simulink model "debugGyros"  (Simulink 9.0)
settings: Solver=FixedStepDiscrete  StartTime=0.0  StopTime=inf  FixedStep=0.01  RelTol=1e-3  EnableMultiTasking=on
InitFcn:
  | ROBOT_DOF=23;
libraries: WBToolboxLibrary x9
settings Model: SuppressorTable=22 serialization::archive 11 0 6 0 0 0 11 0  Creator=DanielePucci  LastModifiedBy=icub
settings DataIOCC: LimitDataPoints=on  SaveFormat=StructureWithTime
settings DebuggingCC: UnderspecifiedInitializationDetection=Simplified  MergeDetectMultiDrivingBlocksExec=error
settings HardwareCC: ProdBitPerPointer=64  ProdLargestAtomicFloat=Float  ProdIntDivRoundTo=Zero  ProdEndianess=LittleEndian  ProdHWDeviceType=Specified

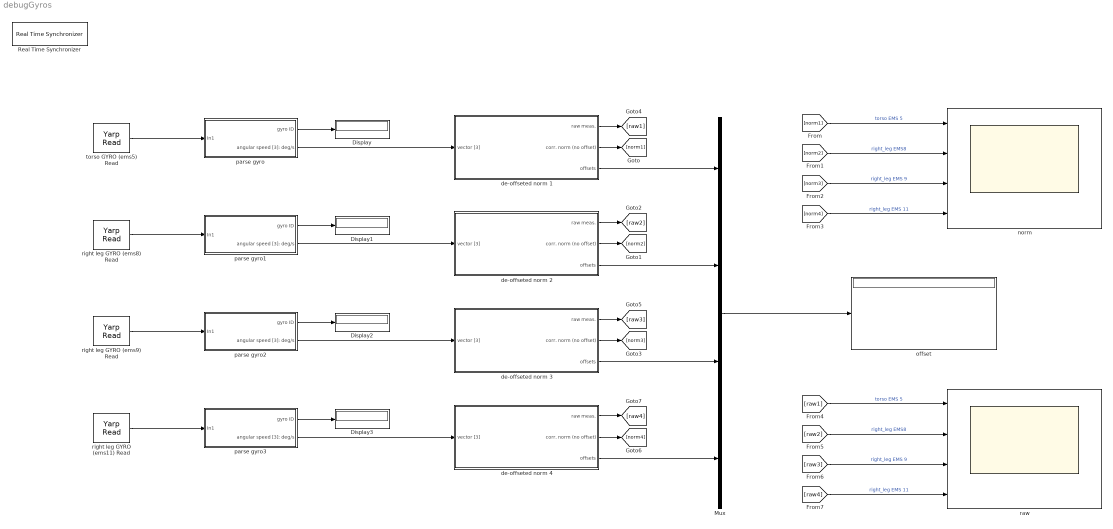
== system debugGyros ==
  Display{,1..3} (4 alike) : Display
  Mux : Mux
  Real Time Synchronizer : WBToolboxLibrary/Utilities/Real Time Synchronizer  period=0.01
      settings: SourceProductName=Whole Body Toolbox
  de-offseted norm 1 : Subsystem
  de-offseted norm 2 : Subsystem
  de-offseted norm 3 : Subsystem
  de-offseted norm 4 : Subsystem
  "norm " : Scope  NumInputPorts=4
  offset : Display
  parse gyro : Subsystem
  parse gyro1 : Subsystem
  parse gyro2 : Subsystem
  parse gyro3 : Subsystem
  raw : Scope  NumInputPorts=4
  right leg GYRO (ems11) Read : WBToolboxLibrary/Utilities/Yarp Read  portName='/icub/right_leg/inertialMTB'  signalSize=86  blocking=off  timestamp=off  autoconnect=on  errorOnConnection=off
      settings: SourceProductName=Whole Body Toolbox
  right leg GYRO (ems8) Read : WBToolboxLibrary/Utilities/Yarp Read  portName='/icub/right_leg/inertialEMS8'  signalSize=8  blocking=off  timestamp=off  autoconnect=on  errorOnConnection=off
      settings: SourceProductName=Whole Body Toolbox
  right leg GYRO (ems9) Read : WBToolboxLibrary/Utilities/Yarp Read  portName='/icub/right_leg/inertialEMS9'  signalSize=8  blocking=off  timestamp=off  autoconnect=on  errorOnConnection=off
      settings: SourceProductName=Whole Body Toolbox
  torso GYRO (ems5) Read : WBToolboxLibrary/Utilities/Yarp Read  portName='/icub/torso/inertialEMS5'  signalSize=8  blocking=off  timestamp=off  autoconnect=on  errorOnConnection=off
      settings: SourceProductName=Whole Body Toolbox
  wires:
  torso GYRO (ems5) Read/1 -> parse gyro/1(In1)
  parse gyro/2(angular speed [3]: deg/s) -> de-offseted norm 1/1(vector [3])
  parse gyro1/2(angular speed [3]: deg/s) -> de-offseted norm 2/1(vector [3])
  right leg GYRO (ems8) Read/1 -> parse gyro1/1(In1)
  parse gyro2/2(angular speed [3]: deg/s) -> de-offseted norm 3/1(vector [3])
  right leg GYRO (ems9) Read/1 -> parse gyro2/1(In1)
  parse gyro3/2(angular speed [3]: deg/s) -> de-offseted norm 4/1(vector [3])
  right leg GYRO (ems11) Read/1 -> parse gyro3/1(In1)
  parse gyro/1(gyro ID) -> Display/1
  parse gyro1/1(gyro ID) -> Display1/1
  parse gyro2/1(gyro ID) -> Display2/1
  parse gyro3/1(gyro ID) -> Display3/1
  de-offseted norm 1/3(offsets) -> Mux/1
  de-offseted norm 2/3(offsets) -> Mux/2
  de-offseted norm 3/3(offsets) -> Mux/3
  de-offseted norm 4/3(offsets) -> Mux/4
  Mux/1 -> offset/1
  de-offseted norm 1/2(corr. norm (no offset)) -> [norm1]
  [norm1] -> "norm "/1  "torso EMS 5"
  [norm2] -> "norm "/2  "right_leg EMS8"
  [norm3] -> "norm "/3  "right_leg EMS 9"
  [norm4] -> "norm "/4  "right_leg EMS 11"
  de-offseted norm 1/1(raw meas.) -> [raw1]
  de-offseted norm 2/1(raw meas.) -> [raw2]
  de-offseted norm 2/2(corr. norm (no offset)) -> [norm2]
  de-offseted norm 3/1(raw meas.) -> [raw3]
  de-offseted norm 3/2(corr. norm (no offset)) -> [norm3]
  de-offseted norm 4/1(raw meas.) -> [raw4]
  de-offseted norm 4/2(corr. norm (no offset)) -> [norm4]
  [raw2] -> raw/2  "right_leg EMS8"
  [raw4] -> raw/4  "right_leg EMS 11"
  [raw1] -> raw/1  "torso EMS 5"
  [raw3] -> raw/3  "right_leg EMS 9"

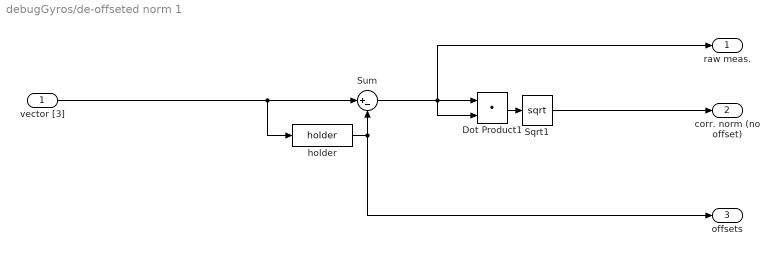
== system debugGyros/de-offseted norm 1 ==
  vector [3] : Inport
  Dot Product1 : DotProduct  InputSameDT=on  OutDataTypeStr=Inherit: Inherit via internal rule
  Sqrt1 : Sqrt  SaturateOnIntegerOverflow=on
  Sum : Sum  Inputs=|+-
  "holder " : WBToolboxLibrary/Utilities/holder 
      settings: SourceProductName=Whole Body Toolbox
  raw meas. : Outport
  corr. norm (no offset) : Outport  Port=2
  offsets : Outport  Port=3
  wires:
  "holder "/1 -> offsets/1, Sum/2
  vector [3]/1 -> "holder "/1, Sum/1
  Dot Product1/1 -> Sqrt1/1
  Sum/1 -> raw meas./1, Dot Product1/2, Dot Product1/1
  Sqrt1/1 -> corr. norm (no offset)/1

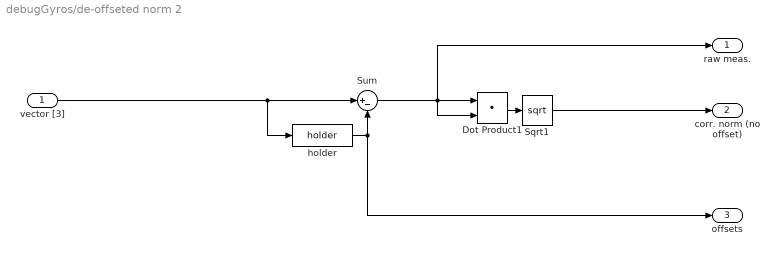
== system debugGyros/de-offseted norm 2 ==
  vector [3] : Inport
  Dot Product1 : DotProduct  InputSameDT=on  OutDataTypeStr=Inherit: Inherit via internal rule
  Sqrt1 : Sqrt  SaturateOnIntegerOverflow=on
  Sum : Sum  Inputs=|+-
  "holder " : WBToolboxLibrary/Utilities/holder 
      settings: SourceProductName=Whole Body Toolbox
  raw meas. : Outport
  corr. norm (no offset) : Outport  Port=2
  offsets : Outport  Port=3
  wires:
  "holder "/1 -> offsets/1, Sum/2
  vector [3]/1 -> "holder "/1, Sum/1
  Dot Product1/1 -> Sqrt1/1
  Sum/1 -> raw meas./1, Dot Product1/2, Dot Product1/1
  Sqrt1/1 -> corr. norm (no offset)/1

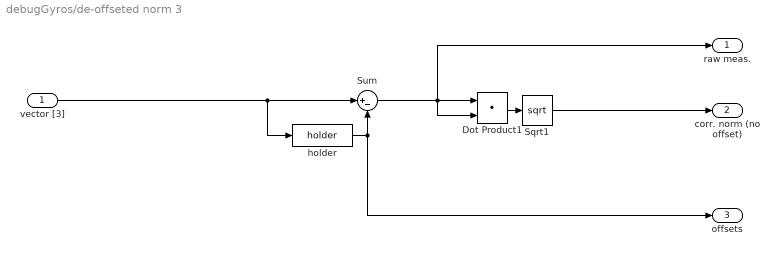
== system debugGyros/de-offseted norm 3 ==
  vector [3] : Inport
  Dot Product1 : DotProduct  InputSameDT=on  OutDataTypeStr=Inherit: Inherit via internal rule
  Sqrt1 : Sqrt  SaturateOnIntegerOverflow=on
  Sum : Sum  Inputs=|+-
  "holder " : WBToolboxLibrary/Utilities/holder 
      settings: SourceProductName=Whole Body Toolbox
  raw meas. : Outport
  corr. norm (no offset) : Outport  Port=2
  offsets : Outport  Port=3
  wires:
  "holder "/1 -> offsets/1, Sum/2
  vector [3]/1 -> "holder "/1, Sum/1
  Dot Product1/1 -> Sqrt1/1
  Sum/1 -> raw meas./1, Dot Product1/2, Dot Product1/1
  Sqrt1/1 -> corr. norm (no offset)/1

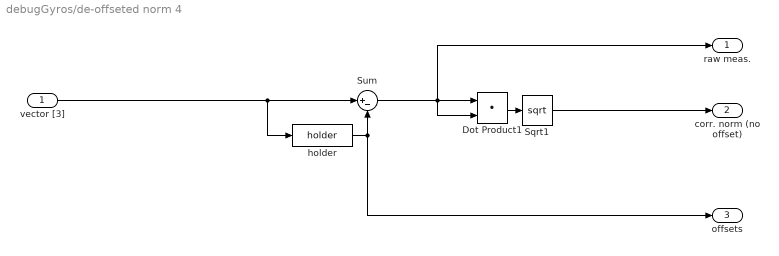
== system debugGyros/de-offseted norm 4 ==
  vector [3] : Inport
  Dot Product1 : DotProduct  InputSameDT=on  OutDataTypeStr=Inherit: Inherit via internal rule
  Sqrt1 : Sqrt  SaturateOnIntegerOverflow=on
  Sum : Sum  Inputs=|+-
  "holder " : WBToolboxLibrary/Utilities/holder 
      settings: SourceProductName=Whole Body Toolbox
  raw meas. : Outport
  corr. norm (no offset) : Outport  Port=2
  offsets : Outport  Port=3
  wires:
  "holder "/1 -> offsets/1, Sum/2
  vector [3]/1 -> "holder "/1, Sum/1
  Dot Product1/1 -> Sqrt1/1
  Sum/1 -> raw meas./1, Dot Product1/2, Dot Product1/1
  Sqrt1/1 -> corr. norm (no offset)/1

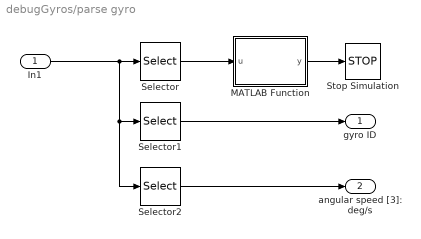
== system debugGyros/parse gyro ==
  In1 : Inport
  MATLAB Function : MATLAB Function  TreatAsAtomicUnit=on
  Selector : Selector  InputPortWidth=8  IndexOptions=Index vector (dialog)  Indices=[1:4]  OutputSizes=1
  Selector1 : Selector  InputPortWidth=8  IndexOptions=Index vector (dialog)  Indices=3  OutputSizes=1
  Selector2 : Selector  InputPortWidth=8  IndexOptions=Index vector (dialog)  Indices=[6 7 8]  OutputSizes=1
  Stop Simulation : Stop
  gyro ID : Outport
  angular speed [3]: deg/s : Outport  Port=2
  wires:
  Selector/1 -> MATLAB Function/1(u)
  Selector1/1 -> gyro ID/1
  Selector2/1 -> angular speed [3]: deg/s/1
  In1/1 -> Selector2/1, Selector1/1, Selector/1
  MATLAB Function/1(y) -> Stop Simulation/1

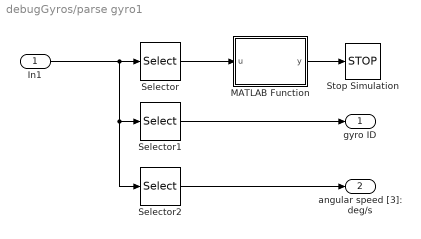
== system debugGyros/parse gyro1 ==
  In1 : Inport
  MATLAB Function : MATLAB Function  TreatAsAtomicUnit=on
  Selector : Selector  InputPortWidth=8  IndexOptions=Index vector (dialog)  Indices=[1:4]  OutputSizes=1
  Selector1 : Selector  InputPortWidth=8  IndexOptions=Index vector (dialog)  Indices=3  OutputSizes=1
  Selector2 : Selector  InputPortWidth=8  IndexOptions=Index vector (dialog)  Indices=[6 7 8]  OutputSizes=1
  Stop Simulation : Stop
  gyro ID : Outport
  angular speed [3]: deg/s : Outport  Port=2
  wires:
  Selector/1 -> MATLAB Function/1(u)
  Selector1/1 -> gyro ID/1
  Selector2/1 -> angular speed [3]: deg/s/1
  In1/1 -> Selector2/1, Selector1/1, Selector/1
  MATLAB Function/1(y) -> Stop Simulation/1

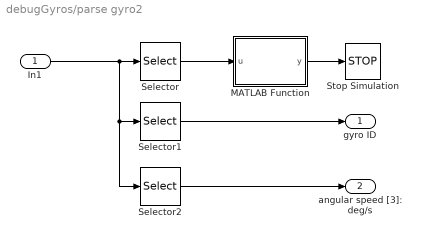
== system debugGyros/parse gyro2 ==
  In1 : Inport
  MATLAB Function : MATLAB Function  TreatAsAtomicUnit=on
  Selector : Selector  InputPortWidth=8  IndexOptions=Index vector (dialog)  Indices=[1:4]  OutputSizes=1
  Selector1 : Selector  InputPortWidth=8  IndexOptions=Index vector (dialog)  Indices=3  OutputSizes=1
  Selector2 : Selector  InputPortWidth=8  IndexOptions=Index vector (dialog)  Indices=[6 7 8]  OutputSizes=1
  Stop Simulation : Stop
  gyro ID : Outport
  angular speed [3]: deg/s : Outport  Port=2
  wires:
  Selector/1 -> MATLAB Function/1(u)
  Selector1/1 -> gyro ID/1
  Selector2/1 -> angular speed [3]: deg/s/1
  In1/1 -> Selector2/1, Selector1/1, Selector/1
  MATLAB Function/1(y) -> Stop Simulation/1

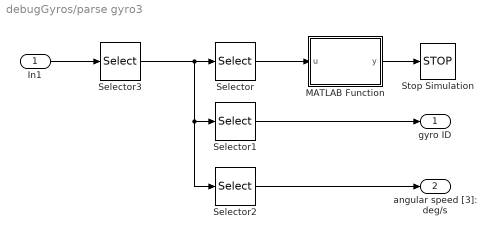
== system debugGyros/parse gyro3 ==
  In1 : Inport
  MATLAB Function : MATLAB Function  TreatAsAtomicUnit=on
  Selector : Selector  InputPortWidth=8  IndexOptions=Index vector (dialog)  Indices=[1:4]  OutputSizes=1
  Selector1 : Selector  InputPortWidth=8  IndexOptions=Index vector (dialog)  Indices=3  OutputSizes=1
  Selector2 : Selector  InputPortWidth=8  IndexOptions=Index vector (dialog)  Indices=[6 7 8]  OutputSizes=1
  Selector3 : Selector  InputPortWidth=86  IndexOptions=Index vector (dialog)  Indices=[1 2 81:86]  OutputSizes=1
  Stop Simulation : Stop
  gyro ID : Outport
  angular speed [3]: deg/s : Outport  Port=2
  wires:
  Selector/1 -> MATLAB Function/1(u)
  Selector1/1 -> gyro ID/1
  Selector2/1 -> angular speed [3]: deg/s/1
  In1/1 -> Selector3/1
  MATLAB Function/1(y) -> Stop Simulation/1
  Selector3/1 -> Selector2/1, Selector1/1, Selector/1

== matlab function parse gyro1/MATLAB Function ==
  data: u input double; y output double
function y = fcn(u)

if (u(1) ~= 1.0 || u(2) ~= 6.0 || u(4) ~= 3.0)
    y = 1;
    error(['Wrong metadata from Gyro ' u(3) '!!']);
else
    y = 0;
end

end

== matlab function parse gyro/MATLAB Function ==
  data: u input double; y output double
function y = fcn(u)

if (u(1) ~= 1.0 || u(2) ~= 6.0 || u(4) ~= 3.0)
    y = 1;
    error(['Wrong metadata from Gyro ' u(3) '!!']);
else
    y = 0;
end

end

== matlab function parse gyro2/MATLAB Function ==
  data: u input double; y output double
function y = fcn(u)

if (u(1) ~= 1.0 || u(2) ~= 6.0 || u(4) ~= 3.0)
    y = 1;
    error(['Wrong metadata from Gyro ' u(3) '!!']);
else
    y = 0;
end

end

== matlab function parse gyro3/MATLAB Function ==
  data: u input double; y output double
function y = fcn(u)

if (u(1) ~= 14.0 || u(2) ~= 6.0 || u(4) ~= 3.0)
    y = 1;
    error(['Wrong metadata from Gyro ' u(3) '!!']);
else
    y = 0;
end

end
